simulink model "W07_S1"  (R2024b)
settings: Solver=ode4  StartTime=0  StopTime=T_final  FixedStep=h  RelTol=1e-3
undefined symbols (not defined in the file or in its folder): a_i, beta_c, h, k_neg, k_pos, k_w, Kb, Kd, Ki, Kp, mp, N_max, N_slow, phi_i, psi_step, rp, T_max, T_min, T_slow, t_step, V_c, w0, w_i, wave_on, x0, X_ff, y_pont, zeta_d, zeta_n
settings Model: Creator=admin  LastModifiedBy=admin
settings DataIOCC: ReturnWorkspaceOutputs=off

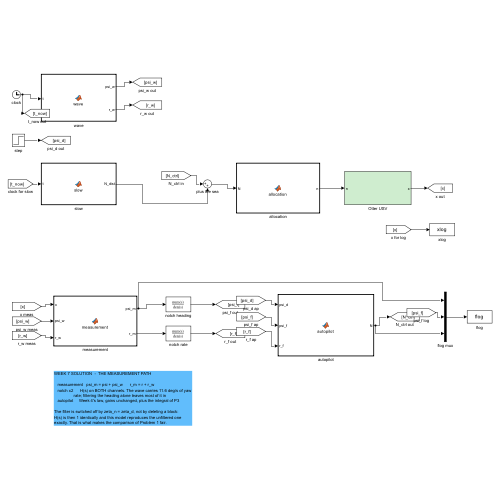
[thumbnail: Simulink's stored preview of the top-level diagram]
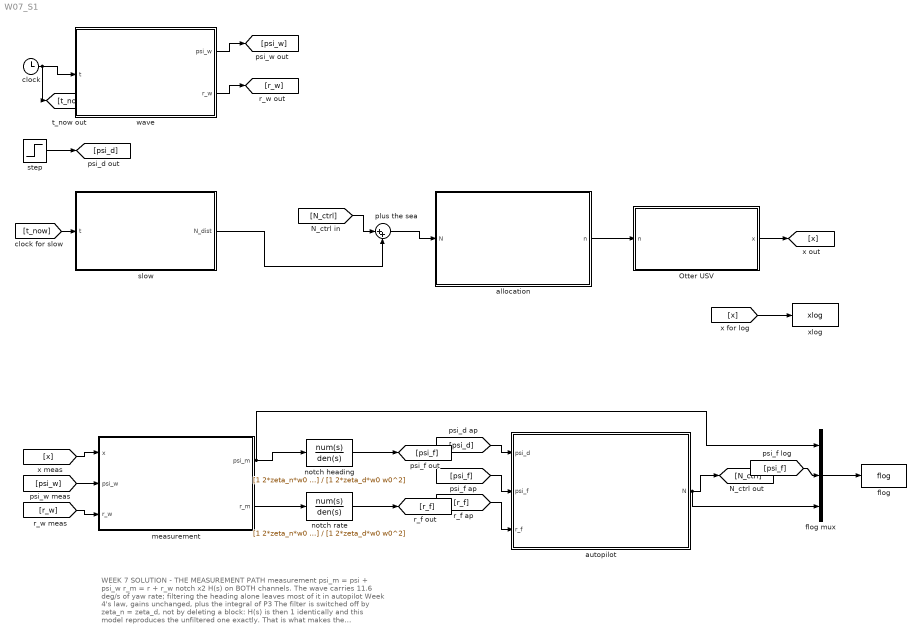
== system W07_S1 ==
  note: WEEK 7 SOLUTION  -  THE MEASUREMENT PATH
      |
      |    measurement   psi_m = psi + psi_w      r_m = r + r_w
      |    notch x2      H(s) on BOTH channels. The wave carries 11.6 deg/s of yaw
      |                  rate; filtering the heading alone leaves most of it in
      |    autopilot     Week 4's law, gains unchanged, plus the integral of P3
      |
      | The filter is switched off by zeta_n = zeta_d, not by deleting a block:
      | H(s) is then 1 identically and this model reproduces the unfiltered one
      | exactly. That is what makes the comparison of Problem 1 fair.
  Otter USV : Subsystem
  allocation : MATLAB Function  TreatAsAtomicUnit=on
  autopilot : MATLAB Function  TreatAsAtomicUnit=on
  clock : Clock
  flog : ToWorkspace  VariableName=flog  SaveFormat=Structure With Time  SampleTime=-1
  flog mux : Mux  Inputs=3
  measurement : MATLAB Function  TreatAsAtomicUnit=on
  notch heading : TransferFcn  Numerator=[1 2*zeta_n*w0 w0^2]  Denominator=[1 2*zeta_d*w0 w0^2]
  notch rate : TransferFcn  Numerator=[1 2*zeta_n*w0 w0^2]  Denominator=[1 2*zeta_d*w0 w0^2]
  plus the sea : Sum  Inputs=|++
  slow : MATLAB Function  TreatAsAtomicUnit=on
  step : Step  Time=t_step  After=psi_step  SampleTime=0
  wave : MATLAB Function  TreatAsAtomicUnit=on
  xlog : ToWorkspace  VariableName=xlog  SaveFormat=Structure With Time  SampleTime=-1
  wires:
  clock/1 -> wave/1(t), [t_now]
  wave/1(psi_w) -> [psi_w]
  wave/2(r_w) -> [r_w]
  step/1 -> [psi_d]
  [t_now] -> slow/1(t)
  [N_ctrl] -> plus the sea/1
  slow/1(N_dist) -> plus the sea/2
  plus the sea/1 -> allocation/1(N)
  allocation/1(n) -> Otter USV/1(n)
  Otter USV/1(x) -> [x]
  [x] -> xlog/1
  [x] -> measurement/1(x)
  [psi_w] -> measurement/2(psi_w)
  [r_w] -> measurement/3(r_w)
  measurement/1(psi_m) -> notch heading/1, flog mux/1
  notch heading/1 -> [psi_f]
  measurement/2(r_m) -> notch rate/1
  notch rate/1 -> [r_f]
  [psi_d] -> autopilot/1(psi_d)
  [psi_f] -> autopilot/2(psi_f)
  [r_f] -> autopilot/3(r_f)
  autopilot/1(N) -> [N_ctrl], flog mux/3
  [psi_f] -> flog mux/2
  flog mux/1 -> flog/1

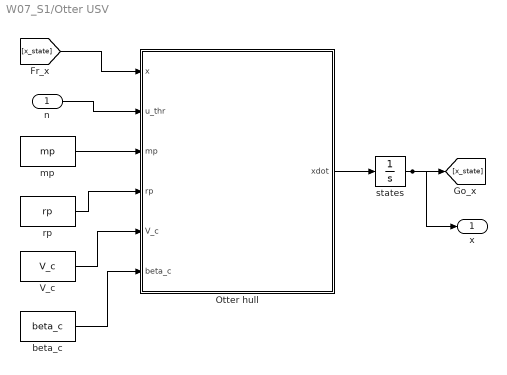
== system W07_S1/Otter USV ==
  n : Inport
  Otter hull : MATLAB Function  TreatAsAtomicUnit=on
  V_c : Constant  Value=V_c
  beta_c : Constant  Value=beta_c
  mp : Constant  Value=mp
  rp : Constant  Value=rp
  states : Integrator  InitialCondition=x0
  x : Outport
  wires:
  n/1 -> Otter hull/2(u_thr)
  [x_state] -> Otter hull/1(x)
  beta_c/1 -> Otter hull/6(beta_c)
  mp/1 -> Otter hull/3(mp)
  states/1 -> [x_state], x/1
  rp/1 -> Otter hull/4(rp)
  Otter hull/1(xdot) -> states/1
  V_c/1 -> Otter hull/5(V_c)

== matlab function W07_S1/slow ==
  data: t input; N_dist output double size=[1 1]; N_slow parameter; T_slow parameter
function N_dist = slow(t, N_slow, T_slow)
%#codegen
%  바람과 2차 파랑 표류를 한 신호로 / wind and second-order drift, as one signal
%
%  파랑(w0 = 3.14 rad/s)보다 두 자리 느리다. 노치는 이것을 **통과시켜야** 한다 —
%  걸러 버리면 제어기가 모르는 사이에 배가 밀려난다.
%  Two decades below the waves. The notch must PASS this: filtered away, the
%  vessel would be pushed off heading without the controller ever seeing it.
N_dist = N_slow*(1 + 0.3*sin(2*pi*t/T_slow));

== matlab function W07_S1/wave ==
  data: t input; psi_w output double size=[1 1]; r_w output; w_i parameter; a_i parameter; phi_i parameter; k_w parameter; wave_on parameter
function [psi_w, r_w] = wave(t, w_i, a_i, phi_i, k_w, wave_on)
%#codegen
%  1차 파랑이 만드는 선수각과 그 변화율 / the wave-induced heading and its rate
%
%      psi_w(t) = k_w sum_i a_i sin(w_i t + phi_i)        [deg]
%      r_w(t)   = k_w sum_i a_i w_i cos(w_i t + phi_i)    [deg/s]
%
%  위상이 정해져 있으므로 이 바다는 매번 똑같다 — 강의의 표를 재현할 수 있다.
%  The phases are fixed, so this sea is the same on every run and the
%  lecture's table can be reproduced.
psi_w = 0;  r_w = 0;
if wave_on ~= 0
    for i = 1:numel(w_i)
        psi_w = psi_w + k_w*a_i(i)*sin(w_i(i)*t + phi_i(i));
        r_w   = r_w   + k_w*a_i(i)*w_i(i)*cos(w_i(i)*t + phi_i(i));
    end
end

== matlab function W07_S1/allocation ==
  data: N input; n output double size=[2 1]; X_ff parameter; y_pont parameter; k_pos parameter; k_neg parameter; T_max parameter; T_min parameter
function n = allocation(N, X_ff, y_pont, k_pos, k_neg, T_max, T_min)
%#codegen
%  6주차의 배분 그대로 / the allocation of Week 6, unchanged
T1 = X_ff/2 + N/(2*y_pont);
T2 = X_ff/2 - N/(2*y_pont);
s = 1;
if T1 > T_max, s = min(s, T_max/T1); end
if T2 > T_max, s = min(s, T_max/T2); end
if T1 < T_min, s = min(s, T_min/T1); end
if T2 < T_min, s = min(s, T_min/T2); end
T1 = s*T1;  T2 = s*T2;
k1 = k_pos;  if T1 < 0, k1 = k_neg; end
k2 = k_pos;  if T2 < 0, k2 = k_neg; end
n = [sign(T1)*sqrt(abs(T1)/k1); sign(T2)*sqrt(abs(T2)/k2)];

== matlab function W07_S1/Otter USV/Otter hull ==
  data: x input; xdot output double size=[12 1]; u_thr input; mp input; rp input; V_c input; beta_c input
function xdot = otter_hull(x, u_thr, mp, rp, V_c, beta_c)
% Fossen's otter.m, called unchanged from Tools/MSS/VESSELS.
%
%   x       12 states, fed back from the integrator
%   u_thr   propeller shaft speeds [rad/s]
%
% otter.m is not written for code generation, so the call is extrinsic and
% xdot has to be pre-sized for Simulink to know the output width.
coder.extrinsic('otter');

xdot = zeros(12,1);
xdot = otter(x, u_thr, mp, rp, V_c, beta_c);
end

== matlab function W07_S1/measurement ==
  data: x input; psi_m output double size=[1 1]; psi_w input; r_w input; r_m output
function [psi_m, r_m] = measurement(x, psi_w, r_w)
%#codegen
%  제어기가 보는 것 = 배가 실제로 하는 것 + 1차 파랑
%  What the controller sees = what the vessel really does + the first-order wave
%
%  센서는 거짓말을 하지 않는다. 배가 정말로 그만큼 흔들리고 있고, 센서는 그것을
%  정직하게 잰다. 문제는 **제어기가 그 흔들림을 오차로 읽는다**는 것이다.
%  The sensor is not lying. The vessel really is oscillating and the sensor
%  reports it truthfully; the trouble is that the controller reads that
%  oscillation as error.
psi_m = x(12)*180/pi + psi_w;    % [deg]
r_m   = x(6)*180/pi  + r_w;      % [deg/s]

== matlab function W07_S1/autopilot ==
  settings: updateMethod=DISCRETE  sampleTime=h
  data: psi_d input; N output double size=[1 1]; psi_f input; r_f input; Kp parameter; Kd parameter; Ki parameter; Kb parameter; N_max parameter; h parameter
function N = autopilot(psi_d, psi_f, r_f, Kp, Kd, Ki, Kb, N_max, h)
%#codegen
%AUTOPILOT  4주차의 법. 게인은 그대로다 — 바뀐 것은 **계측뿐**이다.
%           Week 4's law, gains unchanged; only the measurement is different.
%
%  그것이 이 주차의 요점이다. 파랑을 다루려고 제어기를 다시 튜닝하지 않는다.
%  That is the point of the week: the sea is not answered by retuning.
e = (psi_d - psi_f)*pi/180;
e = atan2(sin(e), cos(e));            % 4주차의 최단각 / the wrap of Week 4
%
%  ── 문제 3: 적분 / the integral of Problem 3 ────────────────────────────
%  느린 외란은 노치를 그대로 통과한다 (§7-6 줄 2). 그러므로 루프가 그것을
%  맞설 수 있고, 맞서려면 오차 없이 맞설 수단 — 적분 — 이 있어야 한다.
%  파랑은 평균이 0 이므로 적분에 쌓이지 않는다. 그래서 노치와 적분이 서로를
%  망치지 않고 함께 산다.
%  The slow push passes the notch untouched, so the loop can oppose it — and
%  opposing it without error needs an integral. The wave has zero mean, so it
%  does not accumulate there: the two coexist.
persistent I
if isempty(I), I = 0; end
u = Kp*e + I - Kd*r_f*pi/180;
N = min(max(u, -N_max), N_max);
%  되감기 방지는 2주차 §2-11 의 back-calculation 그대로
%  Anti-windup by back-calculation, exactly as in Week 2 §2-11
I = I + h*(Ki*e + Kb*(N - u));
